simulink model "gm_uz_mpc_cost_and_optim_state_machine"  (R2021a)
settings: Solver=FixedStepAuto  StartTime=0.0  StopTime=10000*t_ADC  RelTol=1e-3
undefined symbols (not defined in the file or in its folder): A, f, IB, id_ref, iq_ref, ix_ref, iy_ref, lambda_d, lambda_q, lambda_u, lambda_x, lambda_y, Ld_over_LB, Lq_over_LB, n_rpm, omega_m, omegaB, p, psi_pm_over_psiB, Rs_over_ZB, t_ADC, t_clock, Ts_times_ZB_over_Ld, Ts_times_ZB_over_Lq, Ts_times_ZB_over_Lx, Ts_times_ZB_over_Ly, v_dc, VB
libraries: hdlmdlgenlib x73, nesl_utility x38, fl_lib x30, ee_lib x14, simulink x10, hdlsllib x2
(part 1 of 3)
settings Model: Creator=micha  LastModifiedBy=micha
settings SolverCC: AlgebraicLoopSolver=TrustRegion
settings DataIOCC: LimitDataPoints=on  SaveOutput=off  SaveTime=off
settings OptimizationCC: BlockReduction=off  ConditionallyExecuteInputs=off  DefaultParameterBehavior=Inlined  LifeSpan=inf
settings DebuggingCC: AlgebraicLoopMsg=error  InheritedTsInSrcMsg=none  SingleTaskRateTransMsg=error  AllowSymbolicDim=off  StrictBusMsg=ErrorOnBusTreatedAsVector  SFUnexpectedBacktrackingDiag=warning  SFNoUnconditionalDefaultTransitionDiag=warning  SFExecutionAtInitializationDiag=none  SFMachineParentedDataDiag=warning  ArithmeticOperatorsInVariantConditions=warning
settings HardwareCC: ProdBitPerPointer=32  ProdBitPerSizeT=32  ProdBitPerPtrDiffT=32  ProdLargestAtomicFloat=None  ProdIntDivRoundTo=Undefined  ProdEndianess=Unspecified  ProdWordSize=32  ProdHWDeviceType=ASIC/FPGA->ASIC/FPGA  ProdEqTarget=off
settings SFSimCC: SimUseLocalCustomCode=off  CustomCodeUndefinedFunction=UseInterfaceOnly
settings RTWCC: RTWUseLocalCustomCode=off
settings CodeAppCC: StateflowObjectComments=on
settings GRTTargetCC: TargetLangStandard=C89/C90 (ANSI)
settings ConfigComp: CovScope=ReferencedModels  CovMetricSettings=dw  CovSaveCumulativeToWorkspaceVar=on  CovSaveSingleToWorkspaceVar=on  CovExternalEMLEnable=off  CovSFcnEnable=off

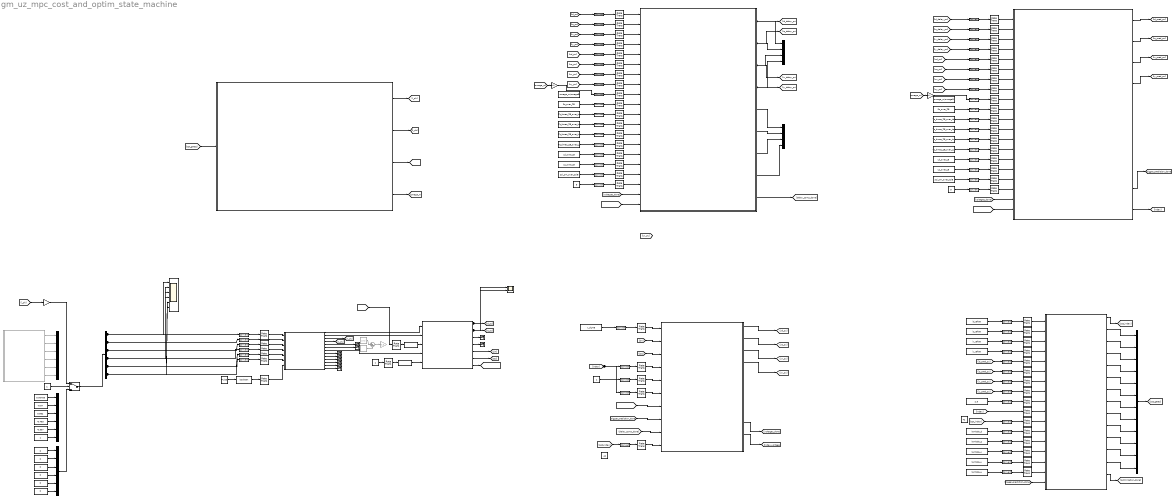
== system gm_uz_mpc_cost_and_optim_state_machine ==
  note: 1=sine source, 2=const
  Constant : Constant  Value=5
  Constant1 : Constant
  Constant10 : Constant  Value=psi_pm_over_psiB
  Constant11 : Constant  Value=2.5
  Constant12 : Constant  Value=42
  Constant13 : Constant  Value=5
  Constant14 : Constant  Value=psi_pm_over_psiB
  Constant15 : Constant  Value=Rs_over_ZB
  Constant16 : Constant  Value=omega_m/omegaB
  Constant17 : Constant  Value=Ts_times_ZB_over_Ld
  Constant18 : Constant  Value=Ts_times_ZB_over_Lq
  Constant19 : Constant  Value=Ts_times_ZB_over_Lx
  Constant2 : Constant  Value=Rs_over_ZB
  Constant20 : Constant  Value=Ts_times_ZB_over_Ly
  Constant21 : Constant  Value=Ld_over_LB
  Constant22 : Constant  Value=Lq_over_LB
  Constant23 : Constant  Value=omega_m/omegaB
  Constant24 : Constant  Commented=on  Value=2*pi
  Constant25 : Constant
  Constant26 : Constant  Value=v_dc/VB
  Constant27 : Constant  Value=iq_ref/IB
  Constant28 : Constant  Value=ix_ref/IB
  Constant29 : Constant  Value=iy_ref/IB
  Constant3 : Constant  Value=Ts_times_ZB_over_Ld
  Constant31 : Constant  Value=lambda_d
  Constant32 : Constant  Value=lambda_q
  Constant33 : Constant  Value=lambda_x
  Constant34 : Constant  Value=lambda_y
  Constant35 : Constant  Value=lambda_u
  Constant36 : Constant  Value=0.00785
  Constant37 : Constant  Value=-0.87
  Constant38 : Constant  Value=0.862
  Constant39 : Constant  Value=-0.493
  Constant4 : Constant  Value=Ts_times_ZB_over_Lq
  Constant40 : Constant  Value=-0.507
  Constant41 : Constant
  Constant42 : Constant  Value=42
  Constant43 : Constant  SampleTime=-1
  Constant{45..50} (6 alike) : Constant  Value=0
  Constant5 : Constant  Value=Ts_times_ZB_over_Lx
  Constant6 : Constant  Value=Ts_times_ZB_over_Ly
  Constant7 : Constant  Value=Ld_over_LB
  Constant8 : Constant  Value=Lq_over_LB
  Constant9 : Constant  Value=id_ref/IB
  Data Type Conversion{,2,31,43,50..51,55..58} (10 alike) : DataTypeConversion  OutDataTypeStr=fixdt_type_xy_currents
  Data Type Conversion{1,5,8,10..11,13,59} (7 alike) : DataTypeConversion  OutDataTypeStr=fixdt_type_polepairs
  Data Type Conversion{12,14..28} (16 alike) : DataTypeConversion  OutDataTypeStr=fixdt_type_constants
  Data Type Conversion29 : DataTypeConversion  OutDataTypeStr=fixdt_type_speed
  Data Type Conversion{3..4,44..45,52..53} (6 alike) : DataTypeConversion  OutDataTypeStr=fixdt_type_dq_currents
  Data Type Conversion30 : DataTypeConversion  OutDataTypeStr=fixdt_type_speed
  Data Type Conversion{32..36,38} (6 alike) : DataTypeConversion  OutDataTypeStr=fixdt_type_vsd
  Data Type Conversion37 : DataTypeConversion  OutDataTypeStr=boolean
  Data Type Conversion39 : DataTypeConversion  OutDataTypeStr=fixdt(1,18,14)
  Data Type Conversion40 : DataTypeConversion  OutDataTypeStr=fixdt_type_voltage
  Data Type Conversion{6..7,41..42,46..49} (8 alike) : DataTypeConversion  OutDataTypeStr=fixdt_type_dqxy_voltages
  Data Type Conversion54 : DataTypeConversion  OutDataTypeStr=fixdt_type_max_current
  Data Type Conversion{60..64} (5 alike) : DataTypeConversion  OutDataTypeStr=fixdt_type_lambda
  Data Type Conversion9 : DataTypeConversion  OutDataTypeStr=fixdt(1,18,14)
  Demux : Demux  Outputs=6
  Gain : Gain  Commented=on  Gain=0.5
  Gain3 : Gain  Gain=1/IB
  Gain4 : Gain  Gain=1/omegaB
  Gain5 : Gain  Gain=1/omegaB
  Mux : Mux
  Mux1 : Mux
  Mux2 : Mux  Inputs=12
  Mux6 : Mux  Inputs=6
  Mux7 : Mux  Inputs=6
  Mux9 : Mux  Inputs=6
  Pulse Generator1 : DiscretePulseGenerator  PulseType=Time based  Period=t_ADC  PulseWidth=5
  Rate Transition{1,5,8..9,60..61} (6 alike) : RateTransition  InitialCondition=1  OutPortSampleTime=t_clock
  Rate Transition{2..4,6..7,10..59,62..66} (60 alike) : RateTransition  OutPortSampleTime=t_clock
  Sawtooth Generator : SignalGenerator  Commented=on  WaveForm=sawtooth  Amplitude=2*pi  Frequency=2*pi*f  Units=rad/sec
  Scope4 : Scope  NumInputPorts=2
  Subsystem : Subsystem  Commented=on
  Subsystem1 : Subsystem
  Sum : Sum  Commented=on  Inputs=|+-
  Switch : Switch  Criteria=u2 > Threshold
  Terminator{,1..9} (10 alike) : Terminator
  natural values : Scope  NumInputPorts=6
  uz_6_ph_mpc_delay_comp : Subsystem  TreatAsAtomicUnit=on
  uz_6ph_mpc_costs_and_optimization : Subsystem  TreatAsAtomicUnit=on
  uz_6ph_mpc_prediction : Subsystem  TreatAsAtomicUnit=on
  uz_6ph_mpc_pu_voltages_vsd : Subsystem  TreatAsAtomicUnit=on
  uz_park_transformation : Subsystem  TreatAsAtomicUnit=on
  uz_vsd_6ph_30deg : Subsystem  TreatAsAtomicUnit=on
  wires:
  [opt_gates] -> Subsystem1/1(In1)
  Subsystem1/4(omega_m) -> [omega_m]
  Subsystem1/3(theta_el) -> [theta_el]
  Subsystem1/2(i_dc) -> [i_dc]
  Subsystem1/1(i_ph) -> [i_ph]
  Constant45/1 -> Mux9/1
  Constant46/1 -> Mux9/2
  Constant48/1 -> Mux9/4
  Constant50/1 -> Mux9/6
  Constant47/1 -> Mux9/3
  Constant49/1 -> Mux9/5
  [omega_m] -> Gain5/1
  [omega_m] -> Gain4/1
  Gain3/1 -> Switch/1
  [opt_index] -> Data Type Conversion10/1
  Constant43/1 -> Switch/2
  Switch/1 -> Demux/1
  [i_ph] -> Gain3/1
  Mux9/1 -> Switch/3
  Constant41/1 -> Mux7/6
  Constant40/1 -> Mux7/5
  Constant39/1 -> Mux7/4
  Constant38/1 -> Mux7/3
  Constant37/1 -> Mux7/2
  Constant36/1 -> Mux7/1
  Subsystem/6(output5) -> Mux6/6
  Subsystem/5(output4) -> Mux6/5
  Subsystem/4(output3) -> Mux6/4
  Subsystem/3(output2) -> Mux6/3
  Subsystem/2(output1) -> Mux6/2
  Subsystem/1(output) -> Mux6/1
  [theta_el] -> Rate Transition38/1
  Demux/5 -> Data Type Conversion36/1, natural values/5
  Demux/3 -> Data Type Conversion34/1, natural values/3
  Demux/6 -> Data Type Conversion38/1, natural values/6
  Demux/1 -> natural values/1, Data Type Conversion32/1
  Demux/4 -> Data Type Conversion35/1, natural values/4
  Demux/2 -> Data Type Conversion33/1, natural values/2
  uz_6ph_mpc_pu_voltages_vsd/4(pu_uy) -> [uy_pu]
  uz_6ph_mpc_pu_voltages_vsd/10(index_voltage) -> [index_voltage]
  [index] -> Data Type Conversion5/1, Data Type Conversion8/1
  [trigger_prediction_done] -> uz_6ph_mpc_costs_and_optimization/17(trigger)
  [trigger_prediction_done] -> uz_6ph_mpc_pu_voltages_vsd/8(trigger_prediction_done)
  [voltages_done] -> uz_6ph_mpc_prediction/19(trigger_voltages_done)
  [delay_comp_done] -> uz_6ph_mpc_pu_voltages_vsd/9(trigger_delay_comp_done)
  [park_done_trigger] -> uz_6_ph_mpc_delay_comp/20(adc_trigger)
  [park_done_trigger] -> uz_6ph_mpc_prediction/20(adc_trigger)
  [park_done_trigger] -> uz_6ph_mpc_pu_voltages_vsd/7(trigger_adc)
  Mux2/1 -> [opt_gates]
  uz_6ph_mpc_costs_and_optimization/13(G11) -> Mux2/12
  uz_6ph_mpc_costs_and_optimization/12(G10) -> Mux2/11
  uz_6ph_mpc_costs_and_optimization/11(G9) -> Mux2/10
  uz_6ph_mpc_costs_and_optimization/10(G8) -> Mux2/9
  uz_6ph_mpc_costs_and_optimization/9(G7) -> Mux2/8
  uz_6ph_mpc_costs_and_optimization/8(G6) -> Mux2/7
  uz_6ph_mpc_costs_and_optimization/7(G5) -> Mux2/6
  uz_6ph_mpc_costs_and_optimization/6(G4) -> Mux2/5
  uz_6ph_mpc_costs_and_optimization/5(G3) -> Mux2/4
  uz_6ph_mpc_costs_and_optimization/4(G2) -> Mux2/3
  uz_6ph_mpc_costs_and_optimization/3(G1) -> Mux2/2
  uz_6ph_mpc_costs_and_optimization/2(G0) -> Mux2/1
  uz_6ph_mpc_costs_and_optimization/14(opt_done) -> [optimization_done]  "optimization done"
  uz_6ph_mpc_costs_and_optimization/1(opt_index) -> [opt_index]  "result"
  Constant35/1 -> Data Type Conversion64/1
  Data Type Conversion64/1 -> Rate Transition66/1
  Rate Transition66/1 -> uz_6ph_mpc_costs_and_optimization/16(lambda_u_AXI)
  Constant34/1 -> Data Type Conversion63/1
  Data Type Conversion63/1 -> Rate Transition65/1
  Rate Transition65/1 -> uz_6ph_mpc_costs_and_optimization/15(lambda_y_AXI)
  Constant33/1 -> Data Type Conversion62/1
  Data Type Conversion62/1 -> Rate Transition64/1
  Rate Transition64/1 -> uz_6ph_mpc_costs_and_optimization/14(lambda_x_AXI)
  Constant32/1 -> Data Type Conversion61/1
  Data Type Conversion61/1 -> Rate Transition63/1
  Rate Transition63/1 -> uz_6ph_mpc_costs_and_optimization/13(lambda_q_AXI)
  Constant31/1 -> Data Type Conversion60/1
  Data Type Conversion60/1 -> Rate Transition62/1
  Rate Transition62/1 -> uz_6ph_mpc_costs_and_optimization/12(lambda_d_AXI)
  Data Type Conversion59/1 -> Rate Transition61/1
  [opt_index] -> Data Type Conversion59/1
  [index] -> Rate Transition60/1
  Rate Transition61/1 -> uz_6ph_mpc_costs_and_optimization/11(last_optim_index)
  Rate Transition60/1 -> uz_6ph_mpc_costs_and_optimization/10(index)
  Data Type Conversion55/1 -> Rate Transition55/1
  Data Type Conversion56/1 -> Rate Transition56/1
  Rate Transition57/1 -> uz_6ph_mpc_costs_and_optimization/1(id_ref_pu_AXI)
  Constant29/1 -> Data Type Conversion56/1
  Rate Transition55/1 -> uz_6ph_mpc_costs_and_optimization/3(ix_ref_pu_AXI)
  Data Type Conversion58/1 -> Rate Transition59/1
  Rate Transition56/1 -> uz_6ph_mpc_costs_and_optimization/4(iy_ref_pu_AXI)
  Rate Transition59/1 -> uz_6ph_mpc_costs_and_optimization/2(iq_ref_pu_AXI)
  Constant28/1 -> Data Type Conversion55/1
  Constant9/1 -> Data Type Conversion57/1
  Constant27/1 -> Data Type Conversion58/1
  Data Type Conversion57/1 -> Rate Transition57/1
  Rate Transition54/1 -> uz_6ph_mpc_costs_and_optimization/9(max_current_pu_AXI)
  Data Type Conversion54/1 -> Rate Transition54/1
  Constant11/1 -> Data Type Conversion54/1
  [iy_pred_pu] -> Data Type Conversion51/1
  [ix_pred_pu] -> Data Type Conversion50/1
  [id_pred_pu] -> Data Type Conversion52/1
  [iq_pred_pu] -> Data Type Conversion53/1
  Data Type Conversion51/1 -> Rate Transition50/1
  Rate Transition53/1 -> uz_6ph_mpc_costs_and_optimization/6(iq_pred_pu)
  Rate Transition50/1 -> uz_6ph_mpc_costs_and_optimization/8(iy_pred_pu)
  Rate Transition51/1 -> uz_6ph_mpc_costs_and_optimization/5(id_pred_pu)
  Rate Transition52/1 -> uz_6ph_mpc_costs_and_optimization/7(ix_pred_pu)
  Data Type Conversion50/1 -> Rate Transition52/1
  Data Type Conversion52/1 -> Rate Transition51/1
  Data Type Conversion53/1 -> Rate Transition53/1
  uz_6ph_mpc_prediction/4(iy_pred_pu) -> [iy_pred_pu]
  uz_6ph_mpc_prediction/3(ix_pred_pu) -> [ix_pred_pu]
  uz_6ph_mpc_prediction/2(iq_pred_pu) -> [iq_pred_pu]
  uz_6ph_mpc_prediction/1(id_pred_pu) -> [id_pred_pu]
  [id_delay_pu] -> Data Type Conversion44/1
  [iq_delay_pu] -> Data Type Conversion45/1
  [ix_delay_pu] -> Data Type Conversion31/1
  [iy_delay_pu] -> Data Type Conversion43/1
  [ix_pu] -> Data Type Conversion/1
  [iy_pu] -> Data Type Conversion2/1
  uz_vsd_6ph_30deg/3(x1) -> [ix_pu]
  uz_vsd_6ph_30deg/4(y1) -> [iy_pu]
  [iq_pu] -> Data Type Conversion4/1
  [id_pu] -> Data Type Conversion3/1
  uz_park_transformation/2(y2) -> [iq_pu], Scope4/2
  uz_park_transformation/1(y1) -> [id_pu], Scope4/1
  [sin] -> uz_6ph_mpc_pu_voltages_vsd/2(sin_angle)
  [cos] -> uz_6ph_mpc_pu_voltages_vsd/3(cos_angle)
  uz_park_transformation/6(cos) -> [cos]
  uz_park_transformation/5(sin) -> [sin]
  [uy_pu] -> Data Type Conversion47/1
  [ux_pu] -> Data Type Conversion46/1
  [ux_pu] -> Data Type Conversion41/1
  [uy_pu] -> Data Type Conversion42/1
  uz_6ph_mpc_pu_voltages_vsd/3(pu_ux) -> [ux_pu]
  [uq_pu] -> Data Type Conversion49/1
  [uq_pu] -> Data Type Conversion7/1
  [ud_pu] -> Data Type Conversion48/1
  [ud_pu] -> Data Type Conversion6/1
  [voltages_done] -> uz_6_ph_mpc_delay_comp/19(trigger_voltages_done)
  uz_6ph_mpc_prediction/9(prediction_done) -> [trigger_prediction_done]
  uz_6ph_mpc_prediction/10(index) -> [index]
  uz_6ph_mpc_pu_voltages_vsd/2(pu_uq) -> [uq_pu]
  Rate Transition49/1 -> uz_6ph_mpc_prediction/6(vq_pu)
  Data Type Conversion45/1 -> Rate Transition45/1
  Rate Transition45/1 -> uz_6ph_mpc_prediction/2(iq_pu)
  Rate Transition44/1 -> uz_6ph_mpc_prediction/3(ix_pu)
  Data Type Conversion48/1 -> Rate Transition48/1
  Rate Transition21/1 -> uz_6ph_mpc_prediction/4(iy_pu)
  Data Type Conversion43/1 -> Rate Transition21/1
  Rate Transition47/1 -> uz_6ph_mpc_prediction/8(vy_pu)
  Data Type Conversion47/1 -> Rate Transition47/1
  Rate Transition46/1 -> uz_6ph_mpc_prediction/7(vx_pu)
  Rate Transition25/1 -> uz_6ph_mpc_prediction/1(id_pu)
  Data Type Conversion49/1 -> Rate Transition49/1
  Data Type Conversion44/1 -> Rate Transition25/1
  Data Type Conversion46/1 -> Rate Transition46/1
  Rate Transition48/1 -> uz_6ph_mpc_prediction/5(vd_pu)
  Data Type Conversion31/1 -> Rate Transition44/1
  Rate Transition14/1 -> uz_6ph_mpc_prediction/14(Ts_times_ZB_over_Ly_AXI)
  Data Type Conversion14/1 -> Rate Transition18/1
  Data Type Conversion17/1 -> Rate Transition14/1
  Rate Transition15/1 -> uz_6ph_mpc_prediction/15(Ld_over_LB_AXI)
  Rate Transition20/1 -> uz_6ph_mpc_prediction/9(omega_m_pu)
  Data Type Conversion30/1 -> Rate Transition20/1
  Rate Transition16/1 -> uz_6ph_mpc_prediction/16(Lq_over_LB_AXI)
  Rate Transition17/1 -> uz_6ph_mpc_prediction/17(psi_pm_over_psiB_AXI)
  Data Type Conversion27/1 -> Rate Transition17/1
  Constant15/1 -> Data Type Conversion12/1
  Constant21/1 -> Data Type Conversion18/1
  Constant17/1 -> Data Type Conversion14/1
  Constant19/1 -> Data Type Conversion16/1
  Data Type Conversion18/1 -> Rate Transition15/1
  Rate Transition19/1 -> uz_6ph_mpc_prediction/12(Ts_times_ZB_over_Lq_AXI)
  Rate Transition12/1 -> uz_6ph_mpc_prediction/13(Ts_times_ZB_over_Lx_AXI)
  Gain5/1 -> Data Type Conversion30/1
  Data Type Conversion16/1 -> Rate Transition12/1
  Data Type Conversion12/1 -> Rate Transition11/1
  Rate Transition18/1 -> uz_6ph_mpc_prediction/11(Ts_times_ZB_over_Ld_AXI)
  Rate Transition11/1 -> uz_6ph_mpc_prediction/10(Rs_over_ZB_AXI)
  Constant18/1 -> Data Type Conversion15/1
  Data Type Conversion19/1 -> Rate Transition16/1
  Data Type Conversion15/1 -> Rate Transition19/1
  Constant22/1 -> Data Type Conversion19/1
  Constant14/1 -> Data Type Conversion27/1
  Constant13/1 -> Data Type Conversion11/1
  Rate Transition10/1 -> uz_6ph_mpc_prediction/18(polepairs_AXI)
  Constant20/1 -> Data Type Conversion17/1
  Data Type Conversion11/1 -> Rate Transition10/1
  uz_park_transformation/7(park_done) -> [park_done_trigger]  "calc_done"
  Rate Transition9/1 -> uz_6ph_mpc_pu_voltages_vsd/10(last_opt_index)
  Data Type Conversion10/1 -> Rate Transition9/1
  Data Type Conversion9/1 -> uz_park_transformation/3(angle_el)
  Constant1/1 -> Data Type Conversion1/1
  Data Type Conversion8/1 -> Rate Transition5/1
  Rate Transition5/1 -> uz_6ph_mpc_pu_voltages_vsd/6(index_AXI)
  Data Type Conversion1/1 -> Rate Transition1/1
  Rate Transition1/1 -> uz_6ph_mpc_pu_voltages_vsd/5(index_select)
  Data Type Conversion5/1 -> Rate Transition8/1
  Rate Transition8/1 -> uz_6ph_mpc_pu_voltages_vsd/4(index)
  uz_6_ph_mpc_delay_comp/9(delay_comp_done) -> [delay_comp_done]
  uz_6_ph_mpc_delay_comp/5(id_delay_pu_AXI) -> Mux1/1
  uz_6_ph_mpc_delay_comp/7(ix_delay_pu_AXI) -> Mux1/3
  uz_6_ph_mpc_delay_comp/8(iy_delay_pu_AXI) -> Mux1/4
  uz_6_ph_mpc_delay_comp/6(iq_delay_pu_AXI) -> Mux1/2
  uz_6_ph_mpc_delay_comp/4(iy_delay_pu) -> Mux/4, [iy_delay_pu]
  uz_6_ph_mpc_delay_comp/3(ix_delay_pu) -> Mux/3, [ix_delay_pu]
  uz_6_ph_mpc_delay_comp/2(iq_delay_pu) -> Mux/2, [iq_delay_pu]
  uz_6_ph_mpc_delay_comp/1(id_delay_pu) -> Mux/1, [id_delay_pu]
  Rate Transition13/1 -> uz_6_ph_mpc_delay_comp/18(polepairs_AXI)
  Data Type Conversion13/1 -> Rate Transition13/1
  Constant/1 -> Data Type Conversion13/1
  Rate Transition28/1 -> uz_6_ph_mpc_delay_comp/17(psi_pm_over_psiB_AXI)
  Data Type Conversion28/1 -> Rate Transition28/1
  Constant10/1 -> Data Type Conversion28/1
  Rate Transition34/1 -> uz_vsd_6ph_30deg/4(a2)
  Data Type Conversion37/1 -> Rate Transition58/1
  Data Type Conversion36/1 -> Rate Transition36/1
  Constant26/1 -> Data Type Conversion40/1
  Data Type Conversion35/1 -> Rate Transition34/1
  uz_vsd_6ph_30deg/5(z1) -> Terminator/1
  Data Type Conversion32/1 -> Rate Transition35/1
  Data Type Conversion33/1 -> Rate Transition32/1
  Rate Transition32/1 -> uz_vsd_6ph_30deg/2(b1)
  Data Type Conversion34/1 -> Rate Transition33/1
  Rate Transition40/1 -> Data Type Conversion39/1
  Constant25/1 -> Rate Transition40/1
  Sawtooth Generator/1 -> Sum/2
  Rate Transition58/1 -> uz_vsd_6ph_30deg/7(pu_conv_valid)
  Sum/1 -> Gain/1
  Rate Transition36/1 -> uz_vsd_6ph_30deg/5(b2)
  Data Type Conversion38/1 -> Rate Transition37/1
  Rate Transition38/1 -> Data Type Conversion9/1
  uz_6ph_mpc_pu_voltages_vsd/1(pu_ud) -> [ud_pu]
  Rate Transition33/1 -> uz_vsd_6ph_30deg/3(c1)
  uz_6ph_mpc_pu_voltages_vsd/9(voltages_done) -> [voltages_done]  "calc_done"
  uz_vsd_6ph_30deg/9(beta_AXI) -> Terminator3/1
  uz_vsd_6ph_30deg/6(z2) -> Terminator1/1
  uz_vsd_6ph_30deg/10(x_AXI) -> Terminator4/1
  Rate Transition37/1 -> uz_vsd_6ph_30deg/6(c2)
  Rate Transition41/1 -> uz_6ph_mpc_pu_voltages_vsd/1(v_DC_pu)
  uz_vsd_6ph_30deg/1(alpha) -> uz_park_transformation/1(u1)
  Data Type Conversion39/1 -> uz_park_transformation/5(factor_angle_el_AXI)
  uz_vsd_6ph_30deg/7(vsd_done) -> uz_park_transformation/4(trigger)
  Pulse Generator1/1 -> Data Type Conversion37/1
  Rate Transition35/1 -> uz_vsd_6ph_30deg/1(a1)
  uz_vsd_6ph_30deg/2(beta) -> uz_park_transformation/2(u2)
  Constant24/1 -> Sum/1
  Data Type Conversion40/1 -> Rate Transition41/1
  uz_vsd_6ph_30deg/11(y_AXI) -> Terminator5/1
  uz_park_transformation/3(y1_AXI) -> Terminator8/1
  uz_vsd_6ph_30deg/13(z2_AXI) -> Terminator7/1
  uz_vsd_6ph_30deg/8(alpha_AXI) -> Terminator2/1
  uz_park_transformation/4(y2_AXI) -> Terminator9/1
  uz_vsd_6ph_30deg/12(z1_AXI) -> Terminator6/1
  Rate Transition43/1 -> uz_6_ph_mpc_delay_comp/8(vy_pu)
  Rate Transition7/1 -> uz_6_ph_mpc_delay_comp/6(vq_pu)
  Rate Transition6/1 -> uz_6_ph_mpc_delay_comp/5(vd_pu)
  Data Type Conversion42/1 -> Rate Transition43/1
  Data Type Conversion7/1 -> Rate Transition7/1
  Data Type Conversion41/1 -> Rate Transition42/1
  Rate Transition42/1 -> uz_6_ph_mpc_delay_comp/7(vx_pu)
  Data Type Conversion6/1 -> Rate Transition6/1
  Rate Transition39/1 -> uz_6_ph_mpc_delay_comp/3(ix_pu)
  Rate Transition4/1 -> uz_6_ph_mpc_delay_comp/2(iq_pu)
  Data Type Conversion2/1 -> Rate Transition2/1
  Data Type Conversion/1 -> Rate Transition39/1
  Data Type Conversion4/1 -> Rate Transition4/1
  Rate Transition3/1 -> uz_6_ph_mpc_delay_comp/1(id_pu)
  Data Type Conversion3/1 -> Rate Transition3/1
  Rate Transition2/1 -> uz_6_ph_mpc_delay_comp/4(iy_pu)
  Rate Transition31/1 -> uz_6_ph_mpc_delay_comp/9(omega_m_pu)
  Gain4/1 -> Data Type Conversion29/1
  Data Type Conversion29/1 -> Rate Transition31/1
  Constant7/1 -> Data Type Conversion25/1
  Constant4/1 -> Data Type Conversion22/1
  Constant5/1 -> Data Type Conversion23/1
  Rate Transition23/1 -> uz_6_ph_mpc_delay_comp/13(Ts_times_ZB_over_Lx_AXI)
  Data Type Conversion20/1 -> Rate Transition22/1
  Rate Transition24/1 -> uz_6_ph_mpc_delay_comp/14(Ts_times_ZB_over_Ly_AXI)
  Rate Transition26/1 -> uz_6_ph_mpc_delay_comp/15(Ld_over_LB_AXI)
  Data Type Conversion23/1 -> Rate Transition23/1
  Data Type Conversion22/1 -> Rate Transition30/1
  Data Type Conversion25/1 -> Rate Transition26/1
  Constant2/1 -> Data Type Conversion20/1
  Constant3/1 -> Data Type Conversion21/1
  Rate Transition27/1 -> uz_6_ph_mpc_delay_comp/16(Lq_over_LB_AXI)
  Rate Transition30/1 -> uz_6_ph_mpc_delay_comp/12(Ts_times_ZB_over_Lq_AXI)
  Constant6/1 -> Data Type Conversion24/1
  Data Type Conversion26/1 -> Rate Transition27/1
  Rate Transition29/1 -> uz_6_ph_mpc_delay_comp/11(Ts_times_ZB_over_Ld_AXI)
  Data Type Conversion21/1 -> Rate Transition29/1
  Rate Transition22/1 -> uz_6_ph_mpc_delay_comp/10(Rs_over_ZB_AXI)
  Constant8/1 -> Data Type Conversion26/1
  Data Type Conversion24/1 -> Rate Transition24/1

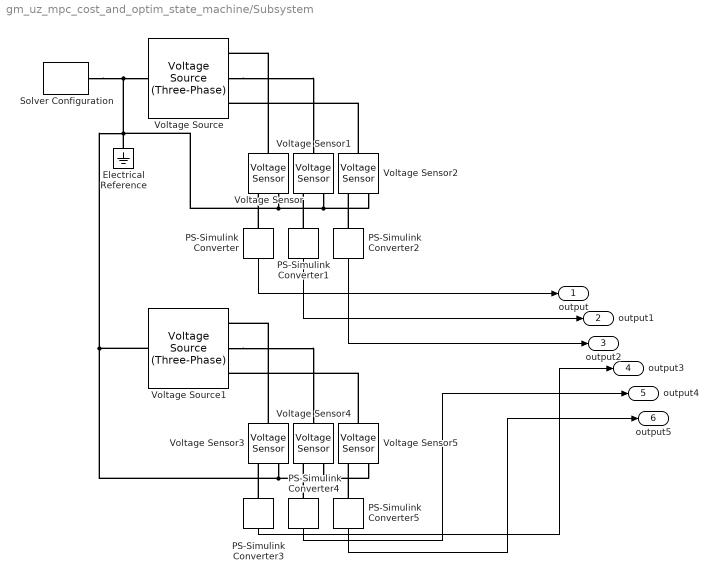
== system gm_uz_mpc_cost_and_optim_state_machine/Subsystem ==
  Electrical Reference : fl_lib/Electrical/Electrical Elements/Electrical Reference
  PS-Simulink Converter{,1..5} (6 alike) : nesl_utility/PS-Simulink Converter  PhysicalDomain=network_engine_domain  SubClassName=ps_output  LeftPortType=input  RightPortType=output  PseudoPeriodic=off  Frequencies=[]  Unit=1  AffineConversion=off
  Solver Configuration : nesl_utility/Solver Configuration  PhysicalDomain=network_engine_domain  SubClassName=solver  LeftPortType=input  RightPortType=generic  Tones=[]  Harmonics=[]  SimulateNoise=off  Profile=off  UseLocalSampling=off  EnableSwitchedLinearOptims=on  FrequencyDomain=off  UseCCode=off  RelTol=0.001  AbsTol=1e-06  MinStep=1e-09  ToWorkspace=off  RevertToSquareIcSolve=off  NumHomotopyIterations=100  PhasorMode=off  PhasorModeNumHarmonics=1  DoDC=off  ResidualTolerance=1e-09  UseLocalSolver=on  LocalSolverChoice=NE_BACKWARD_EULER_ADVANCER  LocalSolverSampleTime=1e-6  DoFixedCost=on  MaxNonlinIter=3  MaxModeIter=2  ComputeImpulses=off  ImpulseIterations=2  LinearAlgebra=Sparse  EquationFormulation=NE_TIME_EF  DelaysMemoryBudget=1024  AutomaticFiltering=on  FilteringTimeConstant=0.001  PartitionStorageMethod=AS_NEEDED  PartitionMemoryBudget=1024  PartitionMethod=FAST
  Voltage Sensor{,1..5} (6 alike) : fl_lib/Electrical/Electrical Sensors/Voltage Sensor
  Voltage Source : ee_lib/Sources/Voltage Source (Three-Phase)  vline_rms=A*sqrt(3)/sqrt(2) V  shift=0 deg  freq=f Hz  impedance_option=1  SShortCircuit=1e6 V*A  XR=15  R=0.01 Ohm  L=3.97e-4 H  G_parasitic=0 1/Ohm  harmonic_option=1  harmonic_orders=Harmonic_Orders  harmonic_ratios=Harmonic_Amplitudes  I_specify=off  I_priority=None  I=[ 0 0 0 ] A  I_nominal_specify=off  I_nominal_unit=A  I_nominal_value=1
      settings: SourceProductBaseCode=PS  InternalSimscapePortConfiguration="{\"Bottom\":[],\"Left\":[{\"id\":\"n\",\"label\":\"n\",\"type\":\"foundation.electrical.electrical\"}],\"Right\":[{\"id\":\"a\",\"label\":\"a\",\"type\":\"foundation.electrical.electrical\"},{\"id\":\"b\",\"label\":\"b\",\"type\":\"foundation.electrical.electrical\"},{\"id\":\"c\",\"label\":\"c\",\"type\":\"foundation.electrical.electrical\"}],\"Top\":[]}"
  Voltage Source1 : ee_lib/Sources/Voltage Source (Three-Phase)  vline_rms=A*sqrt(3)/sqrt(2) V  shift=-30 deg  freq=f Hz  impedance_option=1  SShortCircuit=1e6 V*A  XR=15  R=0.01 Ohm  L=3.97e-4 H  G_parasitic=0 1/Ohm  harmonic_option=1  harmonic_orders=Harmonic_Orders  harmonic_ratios=Harmonic_Amplitudes  I_specify=off  I_priority=None  I=[ 0 0 0 ] A  I_nominal_specify=off  I_nominal_unit=A  I_nominal_value=1
      settings: SourceProductBaseCode=PS  InternalSimscapePortConfiguration="{\"Bottom\":[],\"Left\":[{\"id\":\"n\",\"label\":\"n\",\"type\":\"foundation.electrical.electrical\"}],\"Right\":[{\"id\":\"a\",\"label\":\"a\",\"type\":\"foundation.electrical.electrical\"},{\"id\":\"b\",\"label\":\"b\",\"type\":\"foundation.electrical.electrical\"},{\"id\":\"c\",\"label\":\"c\",\"type\":\"foundation.electrical.electrical\"}],\"Top\":[]}"
  output : Outport
  output1 : Outport  Port=2
  output2 : Outport  Port=3
  output3 : Outport  Port=4
  output4 : Outport  Port=5
  output5 : Outport  Port=6
  wires:
  PS-Simulink Converter2/1 -> output2/1
  PS-Simulink Converter5/1 -> output5/1
  PS-Simulink Converter1/1 -> output1/1
  PS-Simulink Converter4/1 -> output4/1
  PS-Simulink Converter3/1 -> output3/1
  PS-Simulink Converter/1 -> output/1
  connections:
  Voltage Source/RConn2 -- Voltage Sensor1/LConn1
  Voltage Sensor/LConn1 -- Voltage Source/RConn1
  PS-Simulink Converter3/LConn1 -- Voltage Sensor3/RConn1
  PS-Simulink Converter2/LConn1 -- Voltage Sensor2/RConn1
  Voltage Sensor2/LConn1 -- Voltage Source/RConn3
  PS-Simulink Converter4/LConn1 -- Voltage Sensor4/RConn1
  Voltage Sensor5/LConn1 -- Voltage Source1/RConn3
  Voltage Source1/RConn2 -- Voltage Sensor4/LConn1
  PS-Simulink Converter/LConn1 -- Voltage Sensor/RConn1
  Voltage Sensor3/LConn1 -- Voltage Source1/RConn1
  PS-Simulink Converter1/LConn1 -- Voltage Sensor1/RConn1
  PS-Simulink Converter5/LConn1 -- Voltage Sensor5/RConn1
  Voltage Sensor4/RConn2 -- Voltage Sensor3/RConn2 -- Voltage Source1/LConn1 -- Electrical Reference/LConn1 -- Voltage Sensor/RConn2 -- Voltage Sensor1/RConn2 -- Voltage Sensor2/RConn2 -- Voltage Source/LConn1 -- Solver Configuration/RConn1 -- Voltage Sensor5/RConn2

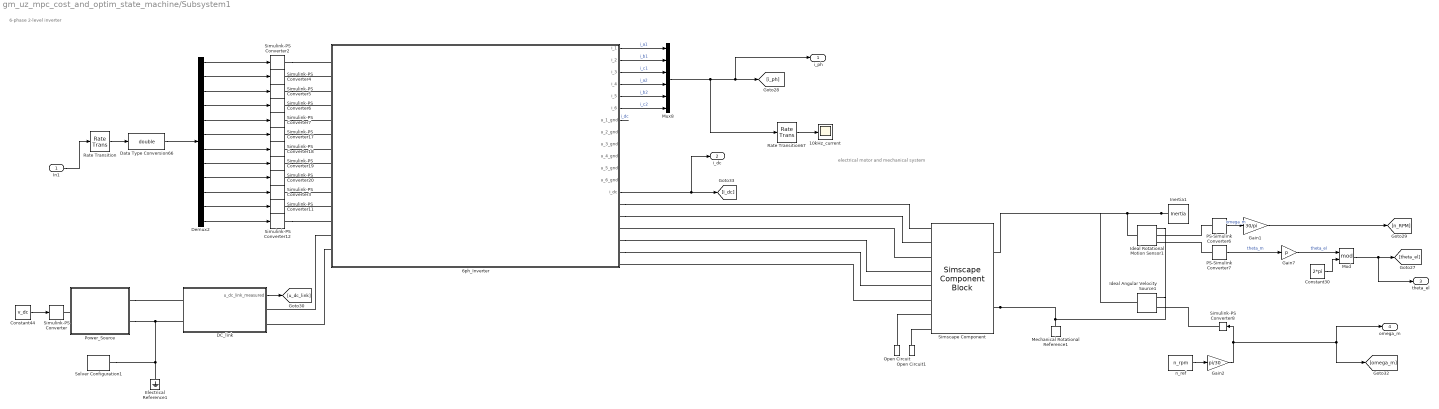
== system gm_uz_mpc_cost_and_optim_state_machine/Subsystem1 ==
  note: 6-phase 2-level inverter
  note: electrical motor and mechanical system
  In1 : Inport
  10kHz_current : Scope
  6ph_Inverter : Subsystem
  Constant30 : Constant  Value=2*pi  SampleTime=-1
  Constant44 : Constant  Value=v_dc  SampleTime=-1
  DC_link : Subsystem
  Data Type Conversion66 : DataTypeConversion  OutDataTypeStr=double
  Demux2 : Demux  Outputs=12
  Electrical Reference1 : fl_lib/Electrical/Electrical Elements/Electrical Reference
  Gain1 : Gain  Gain=30/pi
  Gain2 : Gain  Gain=pi/30
  Gain7 : Gain  Gain=p
  Ideal Angular Velocity Source1 : fl_lib/Mechanical/Mechanical Sources/Ideal Angular Velocity Source
  Ideal Rotational Motion Sensor1 : fl_lib/Mechanical/Mechanical Sensors/Ideal Rotational Motion Sensor  wrap_angle=simscape.enum.onoff.off  offset=0 deg
  Inertia1 : fl_lib/Mechanical/Rotational Elements/Inertia  inertia=J kg*m^2  num_ports=foundation.enum.numPorts2.one  w_specify=off  w_priority=High  w=0 rad/s  w_nominal_specify=off  w_nominal_unit=rad/s  w_nominal_value=1  t_specify=off  t_priority=None  t=0 N*m  t_nominal_specify=off  t_nominal_unit=N*m  t_nominal_value=1
  Mechanical Rotational Reference1 : fl_lib/Mechanical/Rotational Elements/Mechanical Rotational Reference
  Mod : Math  Operator=mod  SaturateOnIntegerOverflow=on
  Mux8 : Mux  Inputs=6
  Open Circuit : fl_lib/Electrical/Electrical Elements/Open Circuit  v_specify=off  v_priority=None  v=0 V  v_nominal_specify=off  v_nominal_unit=V  v_nominal_value=1
      settings: SourceProductBaseCode=SS
  Open Circuit1 : fl_lib/Electrical/Electrical Elements/Open Circuit  v_specify=off  v_priority=None  v=0 V  v_nominal_specify=off  v_nominal_unit=V  v_nominal_value=1
      settings: SourceProductBaseCode=SS
  PS-Simulink Converter6 : nesl_utility/PS-Simulink Converter  PhysicalDomain=network_engine_domain  SubClassName=ps_output  LeftPortType=input  RightPortType=output  PseudoPeriodic=off  Frequencies=[]  Unit=1  AffineConversion=off
      settings: SourceProductBaseCode=PW,SS
  PS-Simulink Converter7 : nesl_utility/PS-Simulink Converter  PhysicalDomain=network_engine_domain  SubClassName=ps_output  LeftPortType=input  RightPortType=output  PseudoPeriodic=off  Frequencies=[]  Unit=1  AffineConversion=off
      settings: SourceProductBaseCode=PW,SS
  Power_Source : Subsystem
  Rate Transition : RateTransition  OutPortSampleTime=1e-6
  Rate Transition67 : RateTransition  OutPortSampleTime=0.0001
  Simscape Component : SimscapeComponentBlock  SourceFile=SixPhase_PMSM  ComponentPath=SixPhase_PMSM  ComponentVariants=SixPhase_PMSM  ComponentVariantNames=SixPhase_PMSM  ClassName=SixPhase_PMSM  SchemaVersion=1  Rs=Rs Ohm  Ld=Ld H  Lq=Lq H  Lx=Lx H  Ly=Ly H  psiPM=psi_pm Wb  np=p  theta_m_specify=off  theta_m_priority=None  theta_m=0 rad  theta_m_nominal_specify=off  theta_m_nominal_unit=rad  theta_m_nominal_value=1
      settings: CopyFcn=simscape.engine.sli.internal.componentblockcallback(gcbh,'COPY')  PreCopyFcn=simscape.engine.sli.internal.componentblockcallback(gcbh,'PRECOPY')  PreDeleteFcn=simscape.engine.sli.internal.componentblockcallback(gcbh,'PREDELETE')  InternalSimscapePortConfiguration="{\"Bottom\":[],\"Left\":[{\"id\":\"a1\",\"label\":\"a1\",\"type\":\"foundation.electrical.electrical\"},{\"id\":\"b1\",\"label\":\"b1\",\"type\":\"foundation.electrical.electrical\"},{\"id\":\"c1\",\"label\":\"c1\",\"type\":\"foundation.electrical.electrical\"},{\"id\":\"a2\",\"label\":\"a2\",\"type\":\"foundation.electrical.electrical\"},{\"id\":\"b2\",\"label\":\"b2\",\"type\":\"foundation.electrical.electrical\"},{\"id\":\"c2\",\"label\":\"c2\",\"type\":\"foundation.electrical.electrical\"},{\"id\":\"n1\",\"label\":\"n1\",\"type\":\"foundation.electrical.electrical\"},{\"id\":\"n2\",\"label\":\"n2\",\"type\":\"foundation.electrical.electrical\"}],\"Right\":[{\"id\":\"R\",\"label\":\"R\",\"type\":\"foundation.mechanical.rotational.rotational\"},{\"id\":\"C\",\"label\":\"C\",\"type\":\"foundation.mechanical.rotational.rotational\"}],\"Top\":[]}"
      mask Type: SixPhase_PMSM
  Simulink-PS Converter{,2..8,11..12,17..20} (14 alike) : nesl_utility/Simulink-PS Converter  PhysicalDomain=network_engine_domain  SubClassName=ps_input  LeftPortType=input  RightPortType=output  PseudoPeriodic=off  Frequencies=[]  NoiseDistribution=none  NoiseParameters=[]  Unit=1  AffineConversion=off  FilteringAndDerivatives=provide  SimscapeFilterOrder=1  InputFilterTimeConstant=0.001  UdotUserProvided=0
      Simulink-PS Converter settings: SourceProductBaseCode=PW,SS
      Simulink-PS Converter8 settings: SourceProductBaseCode=PW,SS
  Solver Configuration1 : nesl_utility/Solver Configuration  PhysicalDomain=network_engine_domain  SubClassName=solver  LeftPortType=input  RightPortType=generic  Tones=[]  Harmonics=[]  SimulateNoise=off  Profile=off  UseLocalSampling=off  EnableSwitchedLinearOptims=on  FrequencyDomain=off  UseCCode=off  RelTol=0.001  AbsTol=1e-06  MinStep=1e-09  ToWorkspace=off  RevertToSquareIcSolve=off  NumHomotopyIterations=100  PhasorMode=off  PhasorModeNumHarmonics=1  DoDC=off  ResidualTolerance=1e-09  UseLocalSolver=on  LocalSolverChoice=NE_BACKWARD_EULER_ADVANCER  LocalSolverSampleTime=1e-6  DoFixedCost=on  MaxNonlinIter=3  MaxModeIter=2  ComputeImpulses=off  ImpulseIterations=2  LinearAlgebra=Sparse  EquationFormulation=NE_TIME_EF  DelaysMemoryBudget=1024  AutomaticFiltering=on  FilteringTimeConstant=0.001  PartitionStorageMethod=AS_NEEDED  PartitionMemoryBudget=1024  PartitionMethod=FAST
      settings: SourceProductBaseCode=PW,SS
  n_ref : Constant  Value=n_rpm  SampleTime=-1
  i_ph : Outport
  i_dc : Outport  Port=2
  theta_el : Outport  Port=3
  omega_m : Outport  Port=4
  wires:
  6ph_Inverter/7(u_1_gnd) -> ?  "i_dc"
  Rate Transition67/1 -> 10kHz_current/1
  Demux2/3 -> Simulink-PS Converter5/1
  n_ref/1 -> Gain2/1
  6ph_Inverter/6(i_6) -> Mux8/6  "i_c2"
  Rate Transition/1 -> Data Type Conversion66/1
  Demux2/8 -> Simulink-PS Converter19/1
  6ph_Inverter/4(i_4) -> Mux8/4  "i_a2"
  Demux2/10 -> Simulink-PS Converter3/1
  Demux2/2 -> Simulink-PS Converter4/1
  Demux2/1 -> Simulink-PS Converter2/1
  Constant44/1 -> Simulink-PS Converter/1
  6ph_Inverter/1(i_1) -> Mux8/1  "i_a1"
  Demux2/7 -> Simulink-PS Converter18/1
  Constant30/1 -> Mod/2
  Demux2/9 -> Simulink-PS Converter20/1
  Demux2/4 -> Simulink-PS Converter6/1
  Demux2/12 -> Simulink-PS Converter12/1
  In1/1 -> Rate Transition/1
  DC_link/1(u_dc_link_measured) -> [u_dc_link]
  6ph_Inverter/2(i_2) -> Mux8/2  "i_b1"
  Mod/1 -> [theta_el], theta_el/1
  Data Type Conversion66/1 -> Demux2/1
  PS-Simulink Converter7/1 -> Gain7/1  "theta_m"
  6ph_Inverter/13(i_dc) -> [i_dc], i_dc/1
  Demux2/5 -> Simulink-PS Converter7/1
  Demux2/6 -> Simulink-PS Converter17/1
  Gain1/1 -> [n_RPM]
  PS-Simulink Converter6/1 -> Gain1/1  "omega_m"
  6ph_Inverter/5(i_5) -> Mux8/5  "i_b2"
  6ph_Inverter/3(i_3) -> Mux8/3  "i_c1"
  Gain7/1 -> Mod/1  "theta_el"
  Gain2/1 -> Simulink-PS Converter8/1, omega_m/1, [omega_m]
  Demux2/11 -> Simulink-PS Converter11/1
  Mux8/1 -> [i_ph], i_ph/1, Rate Transition67/1
  connections:
  Simulink-PS Converter20/RConn1 -- 6ph_Inverter/LConn9
  Simulink-PS Converter2/RConn1 -- 6ph_Inverter/LConn1
  Simulink-PS Converter18/RConn1 -- 6ph_Inverter/LConn7
  6ph_Inverter/RConn1 -- Simscape Component/LConn1
  6ph_Inverter/LConn13 -- DC_link/RConn1
  Power_Source/RConn1 -- DC_link/LConn1
  Simulink-PS Converter8/RConn1 -- Ideal Angular Velocity Source1/RConn1
  Simulink-PS Converter4/RConn1 -- 6ph_Inverter/LConn2
  6ph_Inverter/RConn5 -- Simscape Component/LConn5
  Simulink-PS Converter5/RConn1 -- 6ph_Inverter/LConn3
  PS-Simulink Converter7/LConn1 -- Ideal Rotational Motion Sensor1/RConn3
  Simulink-PS Converter19/RConn1 -- 6ph_Inverter/LConn8
  Simulink-PS Converter/RConn1 -- Power_Source/LConn1
  6ph_Inverter/RConn2 -- Simscape Component/LConn2
  Simscape Component/LConn8 -- Open Circuit1/LConn1
  Simulink-PS Converter7/RConn1 -- 6ph_Inverter/LConn5
  Simscape Component/LConn7 -- Open Circuit/LConn1
  Simulink-PS Converter17/RConn1 -- 6ph_Inverter/LConn6
  6ph_Inverter/RConn4 -- Simscape Component/LConn4
  Simulink-PS Converter12/RConn1 -- 6ph_Inverter/LConn12
  6ph_Inverter/LConn14 -- DC_link/RConn2
  Simscape Component/LConn3 -- 6ph_Inverter/RConn3
  Simulink-PS Converter11/RConn1 -- 6ph_Inverter/LConn11
  Simulink-PS Converter3/RConn1 -- 6ph_Inverter/LConn10
  Simscape Component/RConn2 -- Ideal Angular Velocity Source1/RConn2 -- Ideal Rotational Motion Sensor1/RConn1 -- Mechanical Rotational Reference1/LConn1
  Inertia1/LConn1 -- Ideal Angular Velocity Source1/LConn1 -- Simscape Component/RConn1 -- Ideal Rotational Motion Sensor1/LConn1
  Simscape Component/LConn6 -- 6ph_Inverter/RConn6
  Solver Configuration1/RConn1 -- Power_Source/RConn2 -- DC_link/LConn2 -- Electrical Reference1/LConn1
  PS-Simulink Converter6/LConn1 -- Ideal Rotational Motion Sensor1/RConn2
  Simulink-PS Converter6/RConn1 -- 6ph_Inverter/LConn4

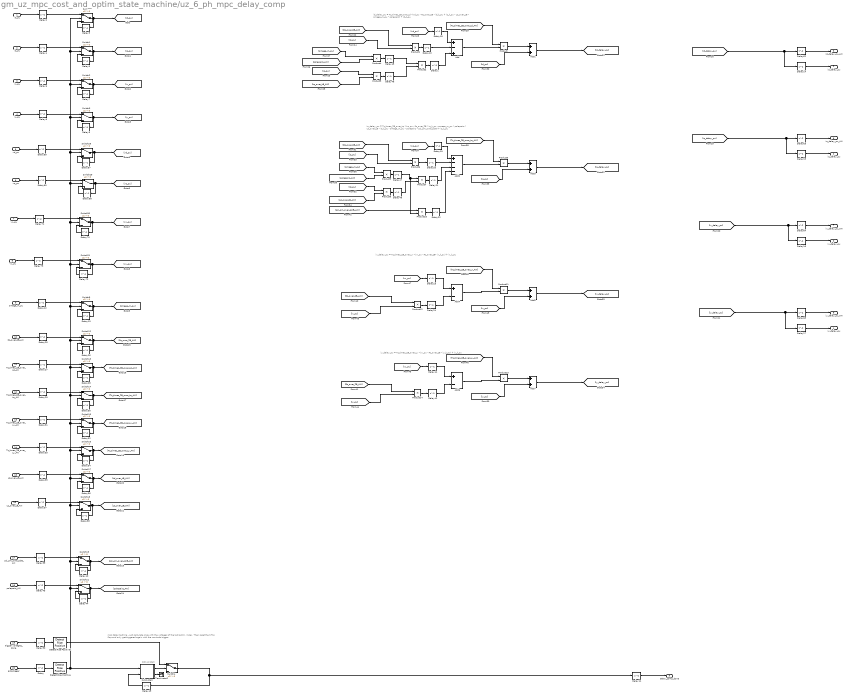
== system gm_uz_mpc_cost_and_optim_state_machine/uz_6_ph_mpc_delay_comp ==
  note: Q=1 at start
  note: id_delay_pu = Ts_times_ZB_over_Ld *(vd_pu - Rs_over_ZB * id_k_pu + iq_k_pu * Lq_over_LB * omega_m_pu * polepairs) + id_k_pu
  note: iq_delay_pu = Ts_times_ZB_over_Lq *(vq_pu - Rs_over_ZB * iq_k_pu - omega_m_pu * polepairs * Ld_over_LB * id_k_pu - omega_m_pu * polepairs * psi_pm_over_psiB) + iq_k_pu
  note: ix_delay_pu = Ts_times_ZB_over_Lx *(vx_pu - Rs_over_ZB* ix_k_pu) + ix_k_pu
  note: iy_delay_pu = Ts_times_ZB_over_Ly *(vy_pu - Rs_over_ZB * iy_k_pu) + iy_k_pu
  note: mpc state machine - just calculate once with the voltages of the last optim. index. Then reset the S flip flop and only
      | get triggered again with the next adc trigger
  id_pu : Inport  OutDataTypeStr=fixdt_type_dq_currents
  iq_pu : Inport  Port=2  OutDataTypeStr=fixdt_type_dq_currents
  ix_pu : Inport  Port=3  OutDataTypeStr=fixdt_type_xy_currents
  iy_pu : Inport  Port=4  OutDataTypeStr=fixdt_type_xy_currents
  vd_pu : Inport  Port=5  OutDataTypeStr=fixdt_type_dqxy_voltages
  vq_pu : Inport  Port=6  OutDataTypeStr=fixdt_type_dqxy_voltages
  vx_pu : Inport  Port=7  OutDataTypeStr=fixdt_type_dqxy_voltages
  vy_pu : Inport  Port=8  OutDataTypeStr=fixdt_type_dqxy_voltages
  omega_m_pu : Inport  Port=9  OutDataTypeStr=fixdt_type_speed
  Rs_over_ZB_AXI : Inport  Port=10  OutDataTypeStr=fixdt_type_constants
  Ts_times_ZB_over_Ld_AXI : Inport  Port=11  OutDataTypeStr=fixdt_type_constants
  Ts_times_ZB_over_Lq_AXI : Inport  Port=12  OutDataTypeStr=fixdt_type_constants
  Ts_times_ZB_over_Lx_AXI : Inport  Port=13  OutDataTypeStr=fixdt_type_constants
  Ts_times_ZB_over_Ly_AXI : Inport  Port=14  OutDataTypeStr=fixdt_type_constants
  Ld_over_LB_AXI : Inport  Port=15  OutDataTypeStr=fixdt_type_constants
  Lq_over_LB_AXI : Inport  Port=16  OutDataTypeStr=fixdt_type_constants
  psi_pm_over_psiB_AXI : Inport  Port=17  OutDataTypeStr=fixdt_type_constants
  polepairs_AXI : Inport  Port=18  OutDataTypeStr=fixdt_type_polepairs
  trigger_voltages_done : Inport  Port=19
  adc_trigger : Inport  Port=20
  Add : Sum  Inputs=+-+  AccumDataTypeStr=fixdt(1,27,16)
  Add{1,3,5,7} (4 alike) : Sum  AccumDataTypeStr=fixdt(1,27,24)
  Add2 : Sum  Inputs=+---  AccumDataTypeStr=fixdt(1,27,16)
  Add4 : Sum  Inputs=+-  AccumDataTypeStr=fixdt(1,27,16)
  Add6 : Sum  Inputs=+-  AccumDataTypeStr=fixdt(1,27,16)
  Delay{,2,4,6,8,11..12,14..17,25,27,29,31,33,35,37,39,43,50,59..60,62..65,71,73} (29 alike) : Delay
  Delay{1,3,5,7,9..10,13,18..24,26,28,30,32,34,36,38,40..42,44..49,57..58,70,72} (34 alike) : Delay  DelayLength=1
  Detect Rise Positive : simulink/Logic and Bit Operations/Detect Rise Positive  vinit=0  OutDataTypeStr=boolean
  Detect Rise Positive1 : simulink/Logic and Bit Operations/Detect Rise Positive  vinit=0  OutDataTypeStr=boolean
  Product{,1..2,4..7,9..14} (13 alike) : Product  OutDataTypeStr=fixdt(1,18,15)
  Product3 : Product  OutDataTypeStr=fixdt(1,27,16)
  Product8 : Product  OutDataTypeStr=fixdt(1,27,16)
  Subsystem : Subsystem
  Switch : Switch  Criteria=u2 > Threshold  OutDataTypeStr=fixdt_type_dq_currents
  Switch1 : Switch  Criteria=u2 > Threshold  OutDataTypeStr=fixdt_type_dq_currents
  Switch{12..19} (8 alike) : Switch  Criteria=u2 > Threshold  OutDataTypeStr=fixdt_type_constants
  Switch2 : Switch  Criteria=u2 > Threshold  OutDataTypeStr=fixdt_type_xy_currents
  Switch21 : Switch  Criteria=u2 > Threshold  OutDataTypeStr=fixdt_type_polepairs
  Switch{28..31} (4 alike) : Switch  Criteria=u2 > Threshold  OutDataTypeStr=fixdt_type_dqxy_voltages
  Switch3 : Switch  Criteria=u2 > Threshold  OutDataTypeStr=fixdt_type_xy_currents
  Switch4 : Switch  Criteria=u2 > Threshold
  Switch5 : Switch  Criteria=u2 > Threshold  OutDataTypeStr=fixdt_type_speed
  Terminator2 : Terminator
  id_delay_pu : Outport
  iq_delay_pu : Outport  Port=2
  ix_delay_pu : Outport  Port=3
  iy_delay_pu : Outport  Port=4
  id_delay_pu_AXI : Outport  Port=5
  iq_delay_pu_AXI : Outport  Port=6
  ix_delay_pu_AXI : Outport  Port=7
  iy_delay_pu_AXI : Outport  Port=8
  delay_comp_done : Outport  Port=9
  wires:
  Detect Rise Positive/1 -> Switch/2, Switch1/2, Switch2/2, Switch3/2, Switch28/2, Switch29/2, Switch30/2, Switch31/2, Switch5/2, Switch12/2, Switch13/2, Switch14/2, Switch15/2, Switch16/2, Switch17/2, Switch18/2, Switch19/2, Switch21/2, Subsystem/1(Set)
  Delay50/1 -> Detect Rise Positive1/1
  trigger_voltages_done/1 -> Delay50/1
  Subsystem/2(!Q) -> Terminator2/1
  Subsystem/1(Q) -> Switch4/2  "Q"
  Detect Rise Positive1/1 -> Switch4/1  "delay_comp done"
  Switch4/1 -> Delay11/1, Delay49/1  "delay_comp_done"
  Delay49/1 -> Subsystem/2(Reset)
  Delay48/1 -> Product7/2
  Product8/1 -> Delay48/1
  Delay47/1 -> Product7/1, Product10/2
  Product9/1 -> Delay47/1
  Delay45/1 -> Product2/1
  Delay46/1 -> Product2/2
  Product3/1 -> Delay46/1
  Product4/1 -> Delay45/1
  Delay41/1 -> Add6/1
  Delay42/1 -> Add6/2
  Product14/1 -> Delay42/1
  [vy_pu] -> Delay41/1  "vy_pu"
  Delay24/1 -> Add4/2
  Product12/1 -> Delay24/1
  Delay23/1 -> Add4/1
  [vx_pu] -> Delay23/1  "vx_pu"
  Product6/1 -> Delay20/1
  Delay19/1 -> Add2/1
  Delay20/1 -> Add2/2
  Delay21/1 -> Add2/3
  Delay22/1 -> Add2/4
  Product10/1 -> Delay22/1
  Product7/1 -> Delay21/1
  [vq_pu] -> Delay19/1  "vq_pu"
  Delay18/1 -> Add/1
  [vd_pu] -> Delay18/1  "vd_pu"
  Delay1/1 -> Add/3
  Delay10/1 -> Add/2
  Product1/1 -> Delay10/1
  Product2/1 -> Delay1/1
  Product13/1 -> Add7/1
  [Ts_times_ZB_over_Ly_AXI] -> Product13/1  "Ts_times_ZB_over_Ly"
  [iy_pu] -> Product14/2  "iy_k_pu"
  [iy_pu] -> Add7/2  "iy_k_pu"
  Add6/1 -> Product13/2
  [Rs_over_ZB_AXI] -> Product14/1  "Rs_over_ZB"
  Product11/1 -> Add5/1
  [ix_pu] -> Add5/2  "ix_k_pu"
  Add4/1 -> Product11/2
  [Rs_over_ZB_AXI] -> Product12/1  "Rs_over_ZB"
  [ix_pu] -> Product12/2  "ix_k_pu"
  [Ts_times_ZB_over_Lx_AXI] -> Product11/1  "Ts_times_ZB_over_Lx"
  [psi_pm_over_psiB_AXI] -> Product10/1
  Product5/1 -> Add3/1
  [polepairs_AXI] -> Product9/2  "polepairs"
  [Ld_over_LB_AXI] -> Product8/2  "Ld_over_LB"
  [id_pu] -> Product8/1  "id_k_pu"
  [iq_pu] -> Add3/2  "iq_k_pu"
  [omega_m_pu] -> Product9/1  "omega_m_pu"
  Add2/1 -> Product5/2
  [Rs_over_ZB_AXI] -> Product6/1  "Rs_over_ZB"
  [iq_pu] -> Product6/2  "iq_k_pu"
  [Ts_times_ZB_over_Lq_AXI] -> Product5/1  "Ts_times_ZB_over_Lq"
  [polepairs_AXI] -> Product4/2  "polepairs"
  [omega_m_pu] -> Product4/1  "omega_m_pu"
  [Lq_over_LB_AXI] -> Product3/2  "Lq_over_LB"
  [iq_pu] -> Product3/1  "iq_k_pu"
  [id_pu] -> Product1/2  "id_k_pu"
  [Rs_over_ZB_AXI] -> Product1/1  "Rs_over_ZB"
  [id_pu] -> Add1/2  "id_k_pu"
  Product/1 -> Add1/1
  [Ts_times_ZB_over_Ld_AXI] -> Product/1  "Ts_times_ZB_over_Ld"
  Add/1 -> Product/2
  Delay17/1 -> iy_delay_pu/1
  Delay16/1 -> ix_delay_pu/1
  Delay14/1 -> id_delay_pu/1
  Delay15/1 -> iq_delay_pu/1
  Delay62/1 -> id_delay_pu_AXI/1
  [ix_delay_pu] -> Delay64/1, Delay16/1
  Delay64/1 -> ix_delay_pu_AXI/1
  Delay65/1 -> iy_delay_pu_AXI/1
  Delay63/1 -> iq_delay_pu_AXI/1
  [id_delay_pu] -> Delay62/1, Delay14/1
  [iq_delay_pu] -> Delay63/1, Delay15/1
  [iy_delay_pu] -> Delay65/1, Delay17/1
  Delay11/1 -> delay_comp_done/1
  Delay30/1 -> Switch14/3
  Delay36/1 -> Switch17/3
  Delay32/1 -> Switch15/3
  Delay13/1 -> Switch5/3
  Delay40/1 -> Switch19/3
  adc_trigger/1 -> Delay/1
  Delay39/1 -> Switch19/1
  Rs_over_ZB_AXI/1 -> Delay25/1
  Delay57/1 -> Switch28/3
  Ts_times_ZB_over_Ld_AXI/1 -> Delay27/1
  Switch1/1 -> Delay5/1, [iq_pu]
  Delay71/1 -> Switch30/1
  Ts_times_ZB_over_Lx_AXI/1 -> Delay31/1
  Switch19/1 -> Delay40/1, [psi_pm_over_psiB_AXI]
  Delay26/1 -> Switch12/3
  Switch18/1 -> [Lq_over_LB_AXI], Delay38/1
  Delay3/1 -> Switch/3
  Ts_times_ZB_over_Lq_AXI/1 -> Delay29/1
  Switch30/1 -> [vx_pu], Delay70/1
  Delay60/1 -> Switch29/1
  Delay70/1 -> Switch30/3
  vy_pu/1 -> Delay73/1
  iy_pu/1 -> Delay8/1
  iq_pu/1 -> Delay4/1
  Lq_over_LB_AXI/1 -> Delay37/1
  Switch5/1 -> Delay13/1, [omega_m_pu]
  vq_pu/1 -> Delay60/1
  Delay27/1 -> Switch13/1
  Delay6/1 -> Switch2/1
  omega_m_pu/1 -> Delay12/1
  Switch31/1 -> [vy_pu], Delay72/1
  Delay73/1 -> Switch31/1
  Delay12/1 -> Switch5/1
  Switch2/1 -> Delay7/1, [ix_pu]
  Delay4/1 -> Switch1/1
  Delay37/1 -> Switch18/1
  Delay7/1 -> Switch2/3
  Ts_times_ZB_over_Ly_AXI/1 -> Delay33/1
  Switch28/1 -> Delay57/1, [vd_pu]
  Delay31/1 -> Switch15/1
  Delay35/1 -> Switch17/1
  Switch/1 -> Delay3/1, [id_pu]
  Switch21/1 -> Delay44/1, [polepairs_AXI]
  id_pu/1 -> Delay2/1
  Delay58/1 -> Switch29/3
  psi_pm_over_psiB_AXI/1 -> Delay39/1
  Delay28/1 -> Switch13/3
  Switch14/1 -> Delay30/1, [Ts_times_ZB_over_Lq_AXI]
  Delay43/1 -> Switch21/1
  Delay72/1 -> Switch31/3
  polepairs_AXI/1 -> Delay43/1
  Switch3/1 -> Delay9/1, [iy_pu]
  Switch29/1 -> Delay58/1, [vq_pu]
  Delay8/1 -> Switch3/1
  Delay29/1 -> Switch14/1
  Delay44/1 -> Switch21/3
  Delay34/1 -> Switch16/3
  Delay/1 -> Detect Rise Positive/1
  Switch13/1 -> Delay28/1, [Ts_times_ZB_over_Ld_AXI]
  Delay9/1 -> Switch3/3
  Switch17/1 -> [Ld_over_LB_AXI], Delay36/1
  Delay38/1 -> Switch18/3
  ix_pu/1 -> Delay6/1
  Switch16/1 -> [Ts_times_ZB_over_Ly_AXI], Delay34/1
  Delay2/1 -> Switch/1
  Ld_over_LB_AXI/1 -> Delay35/1
  Switch15/1 -> Delay32/1, [Ts_times_ZB_over_Lx_AXI]
  vd_pu/1 -> Delay59/1
  vx_pu/1 -> Delay71/1
  Delay33/1 -> Switch16/1
  Delay59/1 -> Switch28/1
  Delay25/1 -> Switch12/1
  Delay5/1 -> Switch1/3
  Add7/1 -> [iy_delay_pu]
  Add1/1 -> [id_delay_pu]
  Add3/1 -> [iq_delay_pu]
  Switch12/1 -> Delay26/1, [Rs_over_ZB_AXI]
  Add5/1 -> [ix_delay_pu]
